simulink model "scheme_3B"  (R2021b)
settings: Solver=VariableStepAuto  StartTime=0.0  StopTime=350  RelTol=1e-3
model workspace (MAT data in the model file):
  Ti = 200
settings Model: Creator=valeria  LastModifiedBy=Ivan
settings SolverCC: AlgebraicLoopSolver=TrustRegion
settings DebuggingCC: SFMachineParentedDataDiag=warning

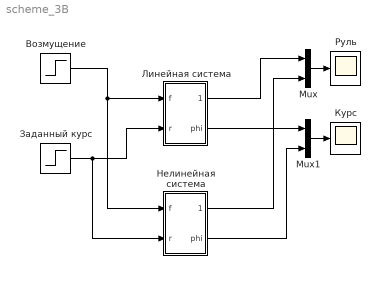
== system scheme_3B ==
  Mux : Mux  Inputs=2
  Mux1 : Mux  Inputs=2
  Возмущение : Step  Time=0  After=0  SampleTime=0.001
  Заданный курс : Step  Time=0  After=90  SampleTime=0.001
  Курс : Scope
  Линейная система : Subsystem
  Нелинейная система : Subsystem
  Руль : Scope
  wires:
  Возмущение/1 -> Нелинейная система/1(f), Линейная система/1(f)
  Заданный курс/1 -> Нелинейная система/2(r), Линейная система/2(r)
  Линейная система/1(delta) -> Mux/1
  Линейная система/2(phi) -> Mux1/1
  Mux/1 -> Руль/1
  Нелинейная система/1(delta) -> Mux/2
  Mux1/1 -> Курс/1
  Нелинейная система/2(phi) -> Mux1/2

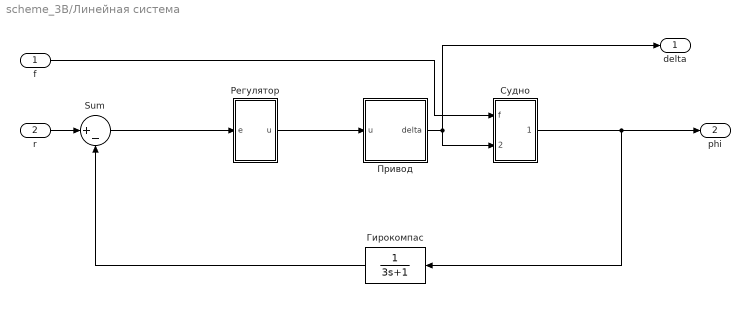
== system scheme_3B/Линейная система ==
  f : Inport
  r : Inport  Port=2
  " Гирокомпас" : TransferFcn  Denominator=[3 1]
  Sum : Sum  Inputs=|+-
  Привод : Subsystem
  Регулятор : Subsystem
  Судно : Subsystem
  delta : Outport
  phi : Outport  Port=2
  wires:
  r/1 -> Sum/1
  Судно/1(phi) -> phi/1, " Гирокомпас"/1
  " Гирокомпас"/1 -> Sum/2
  Привод/1(delta) -> delta/1, Судно/2(delta)
  f/1 -> Судно/1(f)
  Sum/1 -> Регулятор/1(e)
  Регулятор/1(u) -> Привод/1(u)

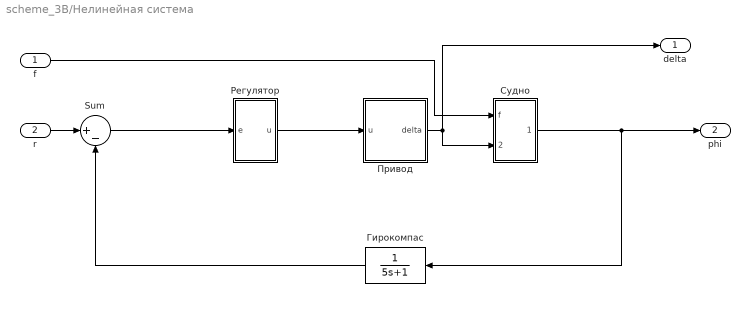
== system scheme_3B/Нелинейная система ==
  f : Inport
  r : Inport  Port=2
  " Гирокомпас" : TransferFcn  Denominator=[5 1]
  Sum : Sum  Inputs=|+-
  Привод : Subsystem
  Регулятор : Subsystem
  Судно : Subsystem
  delta : Outport
  phi : Outport  Port=2
  wires:
  r/1 -> Sum/1
  Судно/1(phi) -> phi/1, " Гирокомпас"/1
  " Гирокомпас"/1 -> Sum/2
  Привод/1(delta) -> delta/1, Судно/2(delta)
  f/1 -> Судно/1(f)
  Sum/1 -> Регулятор/1(e)
  Регулятор/1(u) -> Привод/1(u)

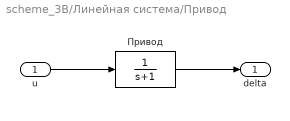
== system scheme_3B/Линейная система/Привод ==
  u : Inport
  Привод : TransferFcn  Denominator=[1 1]
  delta : Outport
  wires:
  Привод/1 -> delta/1
  u/1 -> Привод/1

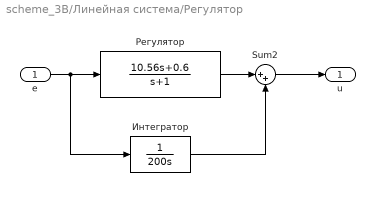
== system scheme_3B/Линейная система/Регулятор ==
  e : Inport
  " Интегратор" : TransferFcn  Denominator=[200 0]
  Sum2 : Sum  Inputs=|++
  Регулятор : TransferFcn  Numerator=[10.56 0.6]  Denominator=[1 1]
  u : Outport
  wires:
  " Интегратор"/1 -> Sum2/2
  e/1 -> " Интегратор"/1, Регулятор/1
  Регулятор/1 -> Sum2/1
  Sum2/1 -> u/1

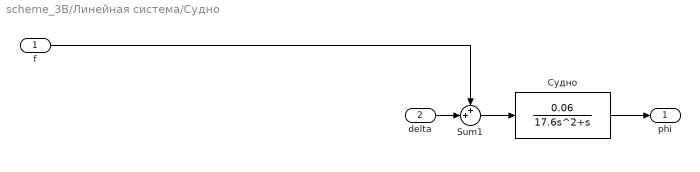
== system scheme_3B/Линейная система/Судно ==
  f : Inport
  delta : Inport  Port=2
  Sum1 : Sum  Inputs=++|
  Судно : TransferFcn  Numerator=[0.06]  Denominator=[17.6 1 0]
  phi : Outport
  wires:
  Sum1/1 -> Судно/1
  Судно/1 -> phi/1
  delta/1 -> Sum1/2
  f/1 -> Sum1/1

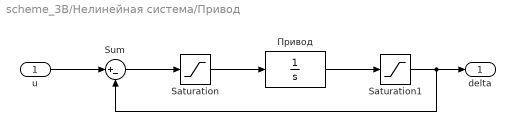
== system scheme_3B/Нелинейная система/Привод ==
  u : Inport
  Saturation : Saturate  UpperLimit=3  LowerLimit=-3
  Saturation1 : Saturate  UpperLimit=30  LowerLimit=-30
  Sum : Sum  Inputs=|+-
  Привод : TransferFcn  Denominator=[1 0]
  delta : Outport
  wires:
  u/1 -> Sum/1
  Sum/1 -> Saturation/1
  Saturation/1 -> Привод/1
  Привод/1 -> Saturation1/1
  Saturation1/1 -> Sum/2, delta/1

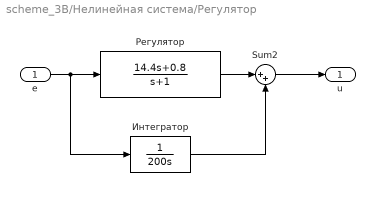
== system scheme_3B/Нелинейная система/Регулятор ==
  e : Inport
  " Интегратор" : TransferFcn  Denominator=[200 0]
  Sum2 : Sum  Inputs=|++
  Регулятор : TransferFcn  Numerator=[14.4 0.8]  Denominator=[1 1]
  u : Outport
  wires:
  " Интегратор"/1 -> Sum2/2
  e/1 -> " Интегратор"/1, Регулятор/1
  Регулятор/1 -> Sum2/1
  Sum2/1 -> u/1

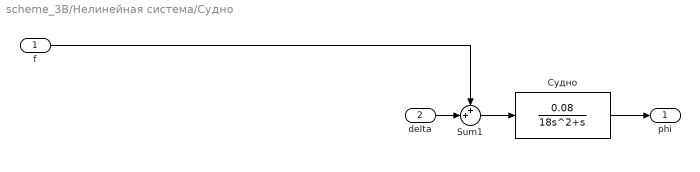
== system scheme_3B/Нелинейная система/Судно ==
  f : Inport
  delta : Inport  Port=2
  Sum1 : Sum  Inputs=++|
  Судно : TransferFcn  Numerator=[0.08]  Denominator=[18 1 0]
  phi : Outport
  wires:
  Sum1/1 -> Судно/1
  Судно/1 -> phi/1
  delta/1 -> Sum1/2
  f/1 -> Sum1/1
